simulink library "thc"  (R2021b)
settings: Solver=VariableStepAuto  StartTime=0.0  StopTime=10.0  RelTol=1e-3
undefined symbols (not defined in the file): ATHC_APTCQA_X_C, ATHC_APTCQB_X_C, ATHC_dAy_X_C, ATHC_Qeq_X_kmh, ATHC_VbaseC_X_C, ATHC_VbaseC_Y_W, ATHC_VbaseD_X_C, ATHC_VbaseH_X_C, FALSE, KTHC_ACMaxMinT_sec, KTHC_aDeice_K, KTHC_AGSDefLv_K, KTHC_AGSLv1_K, KTHC_AGSLv2_K, KTHC_AGSLv3_K, KTHC_AGSLv4_K, KTHC_AGSLv5_K, KTHC_AirIntUpdateT_sec, KTHC_APTCOneZoneMax_W, KTHC_APTCPeriod_cnt, KTHC_APTCPWMEN_flg, KTHC_APTCQMaxC_W, KTHC_APTCQminC_W, KTHC_APTCQminD_W, KTHC_APTCQminRe1_W, KTHC_APTCQminRe_W, KTHC_APTCQoffT_cnt, KTHC_APTCQonT_cnt, KTHC_APTCRiLeMaxDff_W, KTHC_APTCRiLeMinDff_W, KTHC_BatCoolT_cnt, KTHC_BatInTempDef_C, KTHC_bDeice_K, KTHC_CompMaxDeice_rpm, KTHC_CompMinDeice_rpm, KTHC_CompSotxvOp_K, KTHC_CompSotxvOpLow_rpm, KTHC_CompSpdmax_rpm, KTHC_CompSpdmaxBC1_rpm, KTHC_CompSpdmaxBC_rpm, KTHC_CompSpdmid1_rpm, KTHC_CompSpdmid2_rpm, KTHC_CompSpdmid3_rpm, KTHC_CompSpdmid_rpm, KTHC_CompSpdmin_rpm, KTHC_DAPTCQ1_W, KTHC_DAPTCQ2_W, KTHC_DAPTCQ3_W, KTHC_DcChSetTemp_C, KTHC_DehumidityEN_flg, KTHC_DeiceCycTime_K, KTHC_DriveLevelWPTCBAH1_W, KTHC_DriveLevelWPTCBAH2_W, KTHC_DriveLevelWPTCBAH3_W, KTHC_DriveLevelWPTCBAH4_W, KTHC_DriverSeatPos_flg, KTHC_DriveT1MinBAH_C, KTHC_DriveT2MaxBAH_C, KTHC_DriveT2MinBAH_C, KTHC_DriveT3MaxBAH_C ... (+379)
libraries: simulink x489
(part 5 of 17)

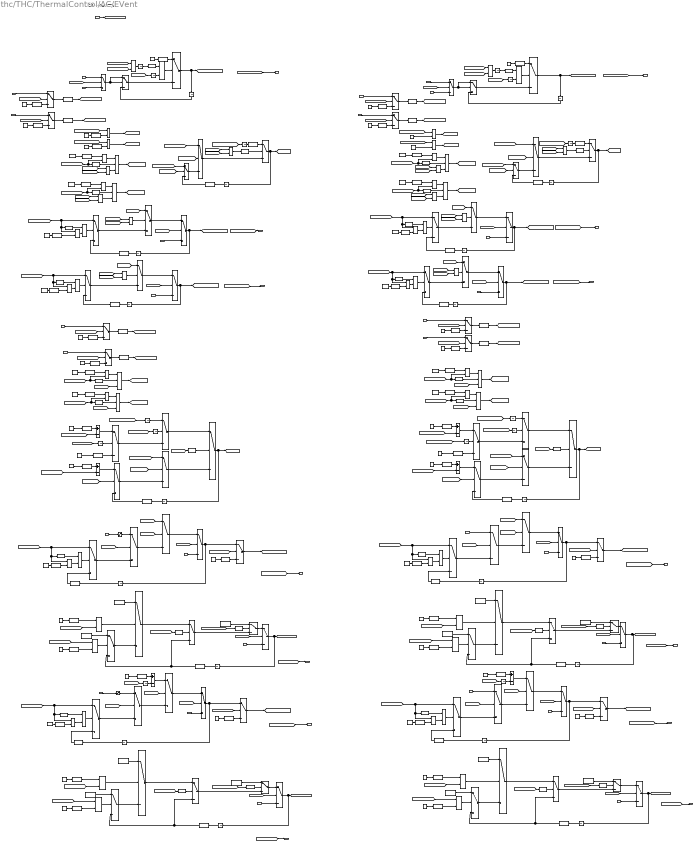
== system thc/THC/ThermalControl/AC/EVent ==
  note: Passenger Side
  note: Driver Side
  fInitial : Inport
  VINP_IVILBlowerModeSta_enum : Inport  Port=2
  VINP_FDCTHCLEventModeStaM_enum : Inport  Port=3
  VINP_IVIRBlowerModeSta_enum : Inport  Port=4
  VINP_FDCTHCREventModeStaM_enum : Inport  Port=5
  VINP_IVILBlowerZSta_enum : Inport  Port=6
  VINP_IVICLBlowerZSta_enum : Inport  Port=7
  VINP_IVIRBlowerZSta_enum : Inport  Port=8
  VINP_IVICRBlowerZSta_enum : Inport  Port=9
  VINP_FDCTHCLEventZStaM_enum : Inport  Port=10
  VINP_FDCTHCCLEVentZStaM_enum : Inport  Port=11
  VINP_FDCTHCREventZStaM_enum : Inport  Port=12
  VINP_FDCTHCCREVentZStaM_enum : Inport  Port=13
  VINP_IVILBlowerYSta_enum : Inport  Port=14
  VINP_IVICLBlowerYSta_enum : Inport  Port=15
  VINP_ZFRTHCLEventActYSta_enum : Inport  Port=16
  VTHC_FDCTHCLVentENM_flg : Inport  Port=17
  VINP_FDCTHCLEventYStaM_enum : Inport  Port=18
  VINP_ZFRTHCCLEVentActYSta_enum : Inport  Port=19
  VTHC_FDCTHCCLVentENM_flg : Inport  Port=20
  VINP_FDCTHCCLEVentYStaM_enum : Inport  Port=21
  VINP_IVIRBlowerYSta_enum : Inport  Port=22
  VINP_IVICRBlowerYSta_enum : Inport  Port=23
  VINP_ZFRTHCREventActYSta_enum : Inport  Port=24
  VTHC_FDCTHCRVentENM_flg : Inport  Port=25
  VINP_FDCTHCREventYStaM_enum : Inport  Port=26
  VINP_ZFRTHCCREVentActYSta_enum : Inport  Port=27
  VTHC_FDCTHCCRVentENM_flg : Inport  Port=28
  VINP_FDCTHCCREVentYStaM_enum : Inport  Port=29
  VINP_CANMsgValidIVI2_flg : Inport  Port=30
  Add{,1..5} (6 alike) : Sum  Inputs=+-
  Constant{,1,4..5,7..8,10,14,18,23,25,28..29,33,38,40..42,45..46,48..51,53..54} (26 alike) : Constant  Value=100
  Constant11 : Constant  Value=3
  Constant12 : Constant  Value=50
  Constant{6,9,13,19,24,34,39,47} (8 alike) : Constant  Value=true
  Constant{15..16,20..21,30..31,35..36} (8 alike) : Constant  Value=126
  Constant{17,22,32,37} (4 alike) : Constant  Value=false
  Constant2 : Constant  Value=2
  Constant26 : Constant  Value=3
  Constant27 : Constant  Value=50
  Constant3 : Constant  Value=2
  Constant43 : Constant
  Constant44 : Constant
  Constant{52,55..61} (8 alike) : Constant  Value=127
  Data Type Conversion{,1..20,22..25,27..35,37..40,42..73} (70 alike) : DataTypeConversion  OutDataTypeStr=uint8
  Data Type Conversion{21,26,36,41} (4 alike) : DataTypeConversion  OutDataTypeStr=boolean
  Detect Change{,1..17,19..20} (20 alike) : simulink/Logic and Bit Operations/Detect Change  vinit=0  OutDataTypeStr=boolean
  Detect Decrease : simulink/Logic and Bit Operations/Detect Decrease  vinit=0.0  OutDataTypeStr=boolean
  Detect Decrease1 : simulink/Logic and Bit Operations/Detect Decrease  vinit=0.0  OutDataTypeStr=boolean
  Detect Increase{,1..7} (8 alike) : simulink/Logic and Bit Operations/Detect Increase  vinit=0.0  OutDataTypeStr=boolean
  Logical Operator{,1..3,5..8} (8 alike) : Logic  Inputs=3  AllPortsSameDT=off  OutDataTypeStr=boolean
  Logical Operator{9..12,22..29} (12 alike) : Logic  AllPortsSameDT=off  OutDataTypeStr=boolean
  Logical Operator{4,13..21} (10 alike) : Logic  Operator=OR  AllPortsSameDT=off  OutDataTypeStr=boolean
  Relational Operator{,1,4..5,7..8,22..23} (8 alike) : RelationalOperator  OutDataTypeStr=boolean  RndMeth=Simplest
  Relational Operator{2,9..10,13,15..16,19,21,24..25,27..28} (12 alike) : RelationalOperator  Operator=<=  OutDataTypeStr=boolean  RndMeth=Simplest
  Relational Operator{3,6,11..12,14,17..18,20} (8 alike) : RelationalOperator  Operator===  OutDataTypeStr=boolean  RndMeth=Simplest
  Saturation : Saturate  UpperLimit=100  LowerLimit=0
  Saturation1 : Saturate  UpperLimit=100  LowerLimit=0
  Switch{,1..81} (82 alike) : Switch  Criteria=u2 > Threshold
  Unit Delay{,1..31} (32 alike) : UnitDelay  SampleTime=-1  HasFrameUpgradeWarning=on
  VTHC_FDCTHCLEventModeSta_enum : Outport
  VTHC_FDCTHCREventModeSta_enum : Outport  Port=2
  VTHC_FDCTHCLEventZSta_enum : Outport  Port=3
  VTHC_FDCTHCCLEVentZSta_enum : Outport  Port=4
  VTHC_FDCTHCREventZSta_enum : Outport  Port=5
  VTHC_FDCTHCCREVentZSta_enum : Outport  Port=6
  VTHC_FDCTHCLEventYSta_enum : Outport  Port=7
  VTHC_FDCTHCLVentEN_flg : Outport  Port=8
  VTHC_FDCTHCCLEVentYSta_enum : Outport  Port=9
  VTHC_FDCTHCCLVentEN_flg : Outport  Port=10
  VTHC_FDCTHCREventYSta_enum : Outport  Port=11
  VTHC_FDCTHCRVentEN_flg : Outport  Port=12
  VTHC_FDCTHCCREVentYSta_enum : Outport  Port=13
  VTHC_FDCTHCCRVentEN_flg : Outport  Port=14
  wires:
  Data Type Conversion73/1 -> Switch81/3
  [VINP_CANMsgValidIVI2_flg] -> Switch81/2
  Switch81/1 -> Data Type Conversion65/1
  VINP_IVICRBlowerYSta_enum/1 -> Switch81/1
  Constant61/1 -> Data Type Conversion73/1
  Constant60/1 -> Data Type Conversion72/1
  VINP_IVIRBlowerYSta_enum/1 -> Switch80/1
  Switch80/1 -> Data Type Conversion64/1
  [VINP_CANMsgValidIVI2_flg] -> Switch80/2
  Data Type Conversion72/1 -> Switch80/3
  VINP_IVICLBlowerYSta_enum/1 -> Switch79/1
  Switch79/1 -> Data Type Conversion63/1
  [VINP_CANMsgValidIVI2_flg] -> Switch79/2
  Constant59/1 -> Data Type Conversion71/1
  Data Type Conversion71/1 -> Switch79/3
  Data Type Conversion70/1 -> Switch78/3
  Constant58/1 -> Data Type Conversion70/1
  [VINP_CANMsgValidIVI2_flg] -> Switch78/2
  Switch78/1 -> Data Type Conversion62/1
  VINP_IVILBlowerYSta_enum/1 -> Switch78/1
  Switch77/1 -> Data Type Conversion61/1
  VINP_IVICRBlowerZSta_enum/1 -> Switch77/1
  [VINP_CANMsgValidIVI2_flg] -> Switch77/2
  Constant57/1 -> Data Type Conversion69/1
  Data Type Conversion69/1 -> Switch77/3
  Data Type Conversion68/1 -> Switch76/3
  Constant56/1 -> Data Type Conversion68/1
  [VINP_CANMsgValidIVI2_flg] -> Switch76/2
  Switch76/1 -> Data Type Conversion60/1
  VINP_IVIRBlowerZSta_enum/1 -> Switch76/1
  VINP_IVICLBlowerZSta_enum/1 -> Switch75/1
  Switch75/1 -> Data Type Conversion59/1
  [VINP_CANMsgValidIVI2_flg] -> Switch75/2
  Constant55/1 -> Data Type Conversion67/1
  Data Type Conversion67/1 -> Switch75/3
  Data Type Conversion66/1 -> Switch74/3
  Constant52/1 -> Data Type Conversion66/1
  [VINP_CANMsgValidIVI2_flg] -> Switch74/2
  Switch74/1 -> Data Type Conversion56/1
  VINP_CANMsgValidIVI2_flg/1 -> [VINP_CANMsgValidIVI2_flg]
  Logical Operator29/1 -> Switch15/2
  [VINP_IVILBlowerZSta_enum] -> Switch12/1, Detect Change13/1, Relational Operator9/1
  Relational Operator9/1 -> Logical Operator28/2
  Detect Change13/1 -> Logical Operator28/1
  Logical Operator28/1 -> Switch12/2
  Logical Operator27/1 -> Switch21/2
  Relational Operator10/1 -> Logical Operator26/2
  [VTHC_FDCTHCCLEVentYSta_enum] -> Add/2
  Constant14/1 -> Data Type Conversion19/1
  Data Type Conversion19/1 -> Add1/1
  [VINP_IVILBlowerYSta_enum] -> Relational Operator13/1
  [fInitial] -> Switch44/2
  VINP_FDCTHCREventYStaM_enum/1 -> Switch58/3
  Constant39/1 -> Switch66/1
  VINP_FDCTHCCREVentYStaM_enum/1 -> Switch67/3
  [VINP_IVICRBlowerYSta_enum] -> Relational Operator23/2, Detect Change9/1
  Relational Operator23/1 -> Logical Operator8/1
  [VTHC_FDCTHCRVentEN_flg] -> Unit Delay26/1
  Data Type Conversion45/1 -> Relational Operator22/1
  Relational Operator7/1 -> Logical Operator5/1
  Detect Change5/1 -> Logical Operator6/2
  Logical Operator6/1 -> [CLYupdate]
  Data Type Conversion21/1 -> Switch32/3, Switch34/3
  VINP_FDCTHCCLEVentYStaM_enum/1 -> Switch44/3
  Switch35/1 -> Switch30/1, Unit Delay11/1
  Switch33/1 -> Switch32/1
  [fInitial] -> Switch35/2
  [VTHC_FDCTHCLVentEN_flg] -> VTHC_FDCTHCLVentEN_flg/1
  Relational Operator14/1 -> Switch42/2
  Switch43/1 -> Switch42/3
  Constant23/1 -> Data Type Conversion29/1
  Logical Operator15/1 -> Switch10/2
  [VTHC_FDCTHCLEventYSta_enum] -> VTHC_FDCTHCLEventYSta_enum/1
  Data Type Conversion23/1 -> Relational Operator12/1
  [fInitial] -> Switch63/2
  Constant26/1 -> Relational Operator17/2
  [VTHC_FDCTHCREventModeSta_enum] -> Relational Operator17/1
  Constant8/1 -> Data Type Conversion7/1
  Data Type Conversion41/1 -> Switch66/3, Switch64/3
  VTHC_FDCTHCCRVentENM_flg/1 -> Switch63/3
  [VTHC_FDCTHCLVentEN_flg] -> Switch30/2
  [LBalanceZ] -> Switch13/1
  [LBalanceMode] -> Detect Increase2/1
  Switch12/1 -> Switch10/3
  Constant19/1 -> Switch34/1
  Logical Operator16/1 -> Switch13/2
  VINP_FDCTHCCLEVentZStaM_enum/1 -> Switch14/3
  Switch15/1 -> Switch13/3
  Switch13/1 -> Switch14/1
  Switch10/1 -> Switch11/1
  Relational Operator18/1 -> Switch56/2
  Relational Operator4/1 -> Logical Operator2/1
  Data Type Conversion62/1 -> [VINP_IVILBlowerYSta_enum]
  Constant5/1 -> Data Type Conversion3/1
  Data Type Conversion3/1 -> Relational Operator5/1
  Constant4/1 -> Data Type Conversion2/1
  Switch28/1 -> Switch27/3
  Detect Change3/1 -> Logical Operator3/2
  Logical Operator3/1 -> [CRZupdate]
  Switch8/1 -> Switch9/3
  Logical Operator2/1 -> [RZupdate]
  [CRZupdate] -> Switch7/2
  Detect Increase1/1 -> Switch9/2
  Switch9/1 -> Unit Delay3/1, [RBalanceZ]
  Unit Delay3/1 -> Data Type Conversion5/1
  Data Type Conversion61/1 -> [VINP_IVICRBlowerZSta_enum]
  [VINP_IVIRBlowerZSta_enum] -> Detect Change2/1, Relational Operator4/2
  Constant7/1 -> Data Type Conversion6/1
  Data Type Conversion11/1 -> Switch15/3
  [LSweepMode] -> Switch28/2
  Switch24/1 -> Switch23/3
  Data Type Conversion9/1 -> Switch9/1
  Unit Delay12/1 -> Data Type Conversion21/1
  Logical Operator5/1 -> [LYupdate]
  Switch48/1 -> Switch47/3
  Switch36/1 -> Switch44/1
  Switch22/1 -> Switch23/1
  Logical Operator13/1 -> Logical Operator1/3
  [VTHC_FDCTHCCREVentZSta_enum] -> VTHC_FDCTHCCREVentZSta_enum/1
  Switch40/1 -> Unit Delay14/1, [VTHC_FDCTHCCLVentEN_flg]
  VTHC_FDCTHCCLVentENM_flg/1 -> Switch40/3
  [LBalanceY] -> Switch27/1
  Data Type Conversion5/1 -> Switch7/3
  [LBalanceMode] -> Switch36/2
  [LSweepMode] -> Switch37/2
  Switch38/1 -> Switch37/3
  Switch37/1 -> Switch36/3
  Switch44/1 -> Unit Delay13/1, Switch39/1
  Data Type Conversion25/1 -> Switch38/3
  Switch39/1 -> [VTHC_FDCTHCCLEVentYSta_enum]
  Switch63/1 -> Unit Delay18/1, [VTHC_FDCTHCCRVentEN_flg]
  Unit Delay13/1 -> Data Type Conversion25/1
  Data Type Conversion4/1 -> Switch4/3
  Switch6/1 -> [LBalanceZ], Unit Delay2/1
  [CRYupdate] -> Switch48/2
  Constant27/1 -> Data Type Conversion32/1
  Data Type Conversion32/1 -> Switch49/3
  Constant32/1 -> Switch56/1
  Unit Delay27/1 -> Switch49/2
  Unit Delay17/1 -> Data Type Conversion40/1
  Switch52/1 -> Switch51/3
  Switch67/1 -> Unit Delay17/1, Switch62/1
  Constant31/1 -> Data Type Conversion37/1
  Data Type Conversion30/1 -> Switch48/3
  Unit Delay15/1 -> Data Type Conversion35/1
  Switch57/1 -> Switch56/3
  [VTHC_FDCTHCCREVentYSta_enum] -> VTHC_FDCTHCCREVentYSta_enum/1
  Data Type Conversion37/1 -> Switch53/3
  Relational Operator21/1 -> Switch66/2
  [VTHC_FDCTHCCRVentEN_flg] -> Switch62/2
  [VINP_IVIRBlowerYSta_enum] -> Relational Operator18/2
  Constant30/1 -> Data Type Conversion38/1
  Constant36/1 -> Data Type Conversion42/1
  [RBalanceY] -> Switch50/1
  Data Type Conversion13/1 -> Switch21/3
  Detect Change10/1 -> Switch55/2
  [RBalanceMode] -> Switch59/2
  Switch54/1 -> Unit Delay16/1, [VTHC_FDCTHCRVentEN_flg]
  Constant33/1 -> Data Type Conversion39/1
  Data Type Conversion33/1 -> Add2/1
  Data Type Conversion6/1 -> Relational Operator7/1
  [RSweepMode] -> Switch60/2
  Switch60/1 -> Switch59/3
  Data Type Conversion40/1 -> Switch61/3
  VINP_ZFRTHCREventActYSta_enum/1 -> Switch51/1
  VTHC_FDCTHCRVentENM_flg/1 -> Switch54/3
  Unit Delay1/1 -> Switch2/3
  VINP_FDCTHCREventModeStaM_enum/1 -> Switch3/3
  fInitial/1 -> [fInitial]
  Detect Change2/1 -> Logical Operator2/2
  [VINP_IVICLBlowerZSta_enum] -> Detect Change1/1, Relational Operator1/2
  [VINP_IVICLBlowerYSta_enum] -> Relational Operator8/2, Detect Change5/1
  Data Type Conversion1/1 -> Relational Operator1/1
  Constant1/1 -> Data Type Conversion1/1
  VINP_ZFRTHCCLEVentActYSta_enum/1 -> Saturation/1
  Constant34/1 -> Switch57/1
  [VINP_IVILBlowerZSta_enum] -> Switch5/1
  [VINP_IVILBlowerYSta_enum] -> Detect Change6/1
  Switch5/1 -> Switch6/3
  Constant/1 -> Data Type Conversion/1
  Detect Change/1 -> Logical Operator/2
  Data Type Conversion26/1 -> Switch43/3, Switch41/3
  [CLZupdate] -> Switch4/2
  Unit Delay18/1 -> Data Type Conversion41/1
  Switch14/1 -> [VTHC_FDCTHCCLEVentZSta_enum], Unit Delay5/1
  Relational Operator17/1 -> [RBalanceMode]
  Unit Delay6/1 -> Data Type Conversion12/1
  [VINP_IVICRBlowerYSta_enum] -> Add3/2
  Unit Delay7/1 -> Data Type Conversion13/1
  Switch18/1 -> Switch16/3
  [VINP_IVICLBlowerYSta_enum] -> Detect Change7/1
  VINP_FDCTHCCREVentZStaM_enum/1 -> Switch20/3
  [fInitial] -> Switch20/2
  [RBalanceMode] -> Logical Operator8/3
  Switch19/1 -> Switch20/1
  Logical Operator20/1 -> Switch19/2
  Switch21/1 -> Switch19/3
  [fInitial] -> Switch11/2
  VINP_ZFRTHCLEventActYSta_enum/1 -> Saturation1/1
  Relational Operator6/1 -> [LSweepMode]
  VINP_FDCTHCLEventModeStaM_enum/1 -> Switch1/3
  Constant20/1 -> Data Type Conversion28/1
  Unit Delay4/1 -> Data Type Conversion10/1
  Switch29/1 -> Switch28/3
  Constant18/1 -> Data Type Conversion24/1
  Logical Operator/1 -> [LZupdate]
  Data Type Conversion60/1 -> [VINP_IVIRBlowerZSta_enum]
  Switch4/1 -> Switch5/3
  Data Type Conversion18/1 -> Add/1
  Switch26/1 -> Switch22/3
  [VTHC_FDCTHCREventZSta_enum] -> Unit Delay9/1
  Relational Operator/1 -> Logical Operator/1
  [VTHC_FDCTHCLEventZSta_enum] -> VTHC_FDCTHCLEventZSta_enum/1
  [CLYupdate] -> Switch25/2
  Unit Delay5/1 -> Data Type Conversion11/1
  Data Type Conversion16/1 -> Switch26/3
  Constant17/1 -> Switch33/1
  Detect Increase3/1 -> Switch46/2
  Unit Delay9/1 -> Data Type Conversion9/1
  [VTHC_FDCTHCCLVentEN_flg] -> Unit Delay24/1
  Data Type Conversion34/1 -> Add3/1
  Detect Change9/1 -> Logical Operator8/2
  Switch62/1 -> [VTHC_FDCTHCCREVentYSta_enum]
  Switch46/1 -> [RBalanceY], Unit Delay19/1
  [VINP_IVIRBlowerYSta_enum] -> Switch47/1
  [VTHC_FDCTHCCRVentEN_flg] -> VTHC_FDCTHCCRVentEN_flg/1
  Add3/1 -> Switch48/1
  [RBalanceMode] -> Logical Operator7/3
  Detect Change6/1 -> Switch32/2
  [VTHC_FDCTHCCREVentYSta_enum] -> Add2/2
  Data Type Conversion28/1 -> Relational Operator14/1
  [fInitial] -> Switch54/2
  Switch50/1 -> Switch58/1
  [RYupdate] -> Switch47/2
  Constant25/1 -> Data Type Conversion33/1
  [VINP_IVICRBlowerZSta_enum] -> Relational Operator5/2, Detect Change3/1
  Switch32/1 -> Switch70/3
  [VINP_IVILBlowerZSta_enum] -> Relational Operator/2, Detect Change/1
  Logical Operator1/1 -> [CLZupdate]
  Data Type Conversion17/1 -> Switch6/1
  [VTHC_FDCTHCLEventZSta_enum] -> Unit Delay10/1
  Data Type Conversion42/1 -> Switch62/3
  [LBalanceZ] -> Switch10/1
  Unit Delay14/1 -> Data Type Conversion26/1
  VINP_IVIRBlowerModeSta_enum/1 -> Switch3/1
  Logical Operator8/1 -> [CRYupdate]
  [VTHC_FDCTHCREventModeSta_enum] -> VTHC_FDCTHCREventModeSta_enum/1
  Constant11/1 -> Data Type Conversion50/1
  Relational Operator13/1 -> Switch34/2
  VINP_IVILBlowerModeSta_enum/1 -> Switch1/1
  Switch1/1 -> Switch/1, Switch/2
  [fInitial] -> Switch3/2
  VTHC_FDCTHCLVentENM_flg/1 -> Switch31/3
  [VTHC_FDCTHCCLEVentZSta_enum] -> VTHC_FDCTHCCLEVentZSta_enum/1
  Switch27/1 -> Switch35/1
  [VTHC_FDCTHCLEventModeSta_enum] -> Relational Operator11/1
  Data Type Conversion24/1 -> Relational Operator13/2
  [VINP_IVICLBlowerYSta_enum] -> Relational Operator15/1
  [fInitial] -> Switch14/2
  Switch25/1 -> Switch24/3
  Unit Delay2/1 -> Data Type Conversion4/1
  Relational Operator1/1 -> Logical Operator1/1
  [VINP_IVILBlowerYSta_enum] -> Switch24/1
  [VINP_IVICRBlowerYSta_enum] -> Relational Operator21/1
  Logical Operator19/1 -> Switch16/2
  VINP_FDCTHCREventZStaM_enum/1 -> Switch17/3
  Detect Change4/1 -> Logical Operator5/2
  [fInitial] -> Switch17/2
  Switch17/1 -> [VTHC_FDCTHCREventZSta_enum], Unit Delay6/1
  [VINP_IVILBlowerYSta_enum] -> Detect Change4/1, Relational Operator7/2
  Switch16/1 -> Switch17/1
  Data Type Conversion20/1 -> Switch29/3
  Data Type Conversion27/1 -> Switch39/3
  [VTHC_FDCTHCREventModeSta_enum] -> Relational Operator3/1
  Constant3/1 -> Relational Operator3/2
  Relational Operator3/1 -> [RSweepMode]
  [VTHC_FDCTHCCLVentEN_flg] -> Switch39/2
  [VTHC_FDCTHCCLEVentYSta_enum] -> VTHC_FDCTHCCLEVentYSta_enum/1
  Constant2/1 -> Data Type Conversion49/1
  [VTHC_FDCTHCLEventModeSta_enum] -> Relational Operator6/1
  [VTHC_FDCTHCRVentEN_flg] -> Switch53/2
  [RBalanceMode] -> Detect Increase3/1
  Switch41/1 -> Switch71/3
  [RSweepMode] -> Switch51/2
  Switch45/1 -> Switch46/1
  Logical Operator7/1 -> [RYupdate]
  Constant12/1 -> Data Type Conversion16/1
  Switch3/1 -> Switch2/2, Switch2/1
  Switch47/1 -> Switch46/3
  Switch11/1 -> Unit Delay4/1, [VTHC_FDCTHCLEventZSta_enum]
  Data Type Conversion35/1 -> Switch52/3
  Switch59/1 -> Switch67/1
  Data Type Conversion7/1 -> Relational Operator8/1
  Detect Change11/1 -> Switch64/2
  Add2/1 -> Switch49/1
  Relational Operator19/1 -> Switch57/2
  [VINP_IVIRBlowerYSta_enum] -> Detect Change8/1, Relational Operator22/2
  [VINP_IVIRBlowerZSta_enum] -> Switch8/1
  Switch53/1 -> [VTHC_FDCTHCREventYSta_enum]
  [VINP_IVIRBlowerYSta_enum] -> Relational Operator19/1
  [fInitial] -> Switch67/2
  Relational Operator22/1 -> Logical Operator7/1
  Switch20/1 -> Unit Delay7/1, [VTHC_FDCTHCCREVentZSta_enum]
  Constant41/1 -> Data Type Conversion46/1
  Constant40/1 -> Data Type Conversion45/1
  [VTHC_FDCTHCLEventModeSta_enum] -> VTHC_FDCTHCLEventModeSta_enum/1
  [VINP_IVICRBlowerZSta_enum] -> Switch7/1
  Unit Delay10/1 -> Data Type Conversion17/1
  Detect Increase/1 -> Switch6/2
  [LZupdate] -> Switch5/2
  Detect Change8/1 -> Logical Operator7/2
  Switch58/1 -> Switch53/1, Unit Delay15/1
  Switch30/1 -> [VTHC_FDCTHCLEventYSta_enum]
  [VTHC_FDCTHCREventYSta_enum] -> Unit Delay31/1
  Add/1 -> Switch26/1
  Detect Change7/1 -> Switch41/2
  [RZupdate] -> Switch8/2
  [fInitial] -> Switch58/2
  Data Type Conversion43/1 -> Relational Operator20/1
  Constant35/1 -> Data Type Conversion43/1
  Relational Operator20/1 -> Switch65/2
  Switch65/1 -> Switch64/1
  Constant38/1 -> Data Type Conversion44/1
  Data Type Conversion46/1 -> Relational Operator23/1
  Data Type Conversion38/1 -> Relational Operator18/1
  [VINP_IVICRBlowerYSta_enum] -> Relational Operator20/2
  [RBalanceMode] -> Switch50/2
  [VTHC_FDCTHCCLVentEN_flg] -> VTHC_FDCTHCCLVentEN_flg/1
  Add1/1 -> Switch25/1
  Unit Delay19/1 -> Data Type Conversion30/1
  Relational Operator15/1 -> Switch43/2
  Switch51/1 -> Switch50/3
  Switch42/1 -> Switch41/1
  Constant24/1 -> Switch43/1
  Data Type Conversion59/1 -> [VINP_IVICLBlowerZSta_enum]
  Unit Delay11/1 -> Data Type Conversion20/1
  Constant15/1 -> Data Type Conversion23/1
  Switch61/1 -> Switch60/3
  [VTHC_FDCTHCREventYSta_enum] -> VTHC_FDCTHCREventYSta_enum/1
  Constant21/1 -> Data Type Conversion27/1
  VINP_FDCTHCLEventZStaM_enum/1 -> Switch11/3
  [RBalanceZ] -> Switch16/1
  Unit Delay16/1 -> Data Type Conversion36/1
  Data Type Conversion14/1 -> Switch25/3
  [VINP_IVILBlowerYSta_enum] -> Relational Operator12/2
  Switch66/1 -> Switch65/3
  Switch56/1 -> Switch55/1
  Unit Delay/1 -> Switch/3
  Constant10/1 -> Data Type Conversion18/1
  Switch49/1 -> Switch45/3
  Switch34/1 -> Switch33/3
  [fInitial] -> Switch31/2
  [RBalanceZ] -> Switch19/1
  [LYupdate] -> Switch24/2
  [VINP_IVICRBlowerYSta_enum] -> Detect Change11/1
  [LBalanceMode] -> Switch27/2
  Relational Operator12/1 -> Switch33/2
  [VINP_IVICLBlowerZSta_enum] -> Switch4/1
  [VINP_IVIRBlowerYSta_enum] -> Detect Change10/1
  Data Type Conversion29/1 -> Relational Operator15/2
  [LBalanceMode] -> Logical Operator5/3
  Detect Change1/1 -> Logical Operator1/2
  [VTHC_FDCTHCRVentEN_flg] -> VTHC_FDCTHCRVentEN_flg/1
  Constant16/1 -> Data Type Conversion22/1
  Data Type Conversion22/1 -> Switch30/3
  Switch7/1 -> Switch8/3
  Data Type Conversion36/1 -> Switch55/3, Switch57/3
  [VINP_IVICLBlowerYSta_enum] -> Relational Operator14/2
  Data Type Conversion12/1 -> Switch18/3
  VINP_IVILBlowerZSta_enum/1 -> Switch74/1
  [fInitial] -> Switch40/2
  Data Type Conversion/1 -> Relational Operator/1
  Data Type Conversion63/1 -> [VINP_IVICLBlowerYSta_enum]
  Switch23/1 -> [LBalanceY], Unit Delay8/1
  Data Type Conversion64/1 -> [VINP_IVIRBlowerYSta_enum]
  Relational Operator8/1 -> Logical Operator6/1
  [VINP_IVICLBlowerYSta_enum] -> Add1/2
  Relational Operator5/1 -> Logical Operator3/1
  Data Type Conversion39/1 -> Relational Operator19/2
  Data Type Conversion44/1 -> Relational Operator21/2
  Switch68/1 -> Unit Delay/1, [VTHC_FDCTHCLEventModeSta_enum]
  VINP_ZFRTHCCREVentActYSta_enum/1 -> Switch60/1
  [VTHC_FDCTHCREventZSta_enum] -> VTHC_FDCTHCREventZSta_enum/1
  Data Type Conversion2/1 -> Relational Operator4/1
  Constant22/1 -> Switch42/1
  [fInitial] -> Switch1/2
  Constant37/1 -> Switch65/1
  Switch31/1 -> [VTHC_FDCTHCLVentEN_flg], Unit Delay12/1
  Data Type Conversion10/1 -> Switch12/3
  Unit Delay8/1 -> Data Type Conversion14/1
  VINP_FDCTHCLEventYStaM_enum/1 -> Switch35/3
  Constant29/1 -> Data Type Conversion34/1
  [LBalanceMode] -> Logical Operator6/3
  [VTHC_FDCTHCCLVentEN_flg] -> Logical Operator9/2
  [VTHC_FDCTHCLVentEN_flg] -> Logical Operator9/1
  Logical Operator9/1 -> Unit Delay20/1
  Unit Delay20/1 -> Detect Decrease/1
  Detect Decrease/1 -> Logical Operator10/1
  Data Type Conversion49/1 -> Relational Operator6/2
  Data Type Conversion50/1 -> Relational Operator11/2
  [LBalanceMode] -> Unit Delay21/1
  Unit Delay21/1 -> Logical Operator10/2
  Logical Operator10/1 -> Switch68/2
  Data Type Conversion51/1 -> Switch68/1
  Constant43/1 -> Data Type Conversion51/1
  Switch/1 -> Switch68/3
  Constant44/1 -> Data Type Conversion52/1
  Data Type Conversion52/1 -> Switch69/1
  Logical Operator11/1 -> Switch69/2
  Detect Decrease1/1 -> Logical Operator11/1
  Unit Delay22/1 -> Detect Decrease1/1
  Logical Operator12/1 -> Unit Delay22/1
  [VTHC_FDCTHCRVentEN_flg] -> Logical Operator12/1
  [VTHC_FDCTHCCRVentEN_flg] -> Logical Operator12/2
  Switch69/1 -> Unit Delay1/1, [VTHC_FDCTHCREventModeSta_enum]
  Switch2/1 -> Switch69/3
  [RBalanceMode] -> Unit Delay23/1
  Unit Delay23/1 -> Logical Operator11/2
  Constant45/1 -> Data Type Conversion53/1
  Data Type Conversion53/1 -> Add4/1
  [LBalanceY] -> Unit Delay28/1
  Add4/1 -> Switch36/1
  Add5/1 -> Switch59/1
  Constant46/1 -> Data Type Conversion54/1
  Data Type Conversion54/1 -> Add5/1
  [RBalanceY] -> Unit Delay30/1
  Logical Operator4/1 -> Logical Operator/3
  [LBalanceMode] -> Logical Operator4/1
  [LSweepMode] -> Logical Operator4/2
  [LSweepMode] -> Logical Operator13/2
  [LBalanceMode] -> Logical Operator13/1
  [LBalanceMode] -> Logical Operator14/1
  [LSweepMode] -> Logical Operator14/2
  Logical Operator14/1 -> Detect Increase/1
  [LBalanceMode] -> Logical Operator15/1
  [LSweepMode] -> Logical Operator15/2
  [LSweepMode] -> Logical Operator16/2
  [LBalanceMode] -> Logical Operator16/1
  Logical Operator17/1 -> Logical Operator2/3
  [RSweepMode] -> Logical Operator17/1
  [RBalanceMode] -> Logical Operator17/2
  [RBalanceMode] -> Logical Operator18/2
  [RSweepMode] -> Logical Operator18/1
  Logical Operator18/1 -> Logical Operator3/3
  [RSweepMode] -> Logical Operator19/1
  [RBalanceMode] -> Logical Operator19/2
  [RBalanceMode] -> Logical Operator20/2
  [RSweepMode] -> Logical Operator20/1
  [RBalanceMode] -> Logical Operator21/2
  [RSweepMode] -> Logical Operator21/1
  Logical Operator21/1 -> Detect Increase1/1
  Switch70/1 -> Switch31/1
  Constant6/1 -> Switch70/1
  Detect Increase5/1 -> Switch70/2
  [LBalanceMode] -> Detect Increase5/1
  [LBalanceMode] -> Detect Increase4/1
  Detect Increase4/1 -> Switch71/2
  Constant47/1 -> Switch71/1
  Switch71/1 -> Switch40/1
  [VTHC_FDCTHCLEventYSta_enum] -> Unit Delay29/1
  Detect Increase2/1 -> Switch23/2
  Saturation/1 -> Switch37/1
  Saturation1/1 -> Switch28/1
  Unit Delay24/1 -> Switch26/2
  [VTHC_FDCTHCLVentEN_flg] -> Unit Delay25/1
  Unit Delay25/1 -> Switch22/2
  Unit Delay26/1 -> Switch45/2
  [VTHC_FDCTHCCRVentEN_flg] -> Unit Delay27/1
  [RBalanceMode] -> Detect Increase7/1
  Detect Increase7/1 -> Switch72/2
  Constant9/1 -> Switch72/1
  Switch55/1 -> Switch72/3
  Switch72/1 -> Switch54/1
  Switch64/1 -> Switch73/3
  Constant13/1 -> Switch73/1
  Detect Increase6/1 -> Switch73/2
  [RBalanceMode] -> Detect Increase6/1
  Switch73/1 -> Switch63/1
  [VINP_IVICLBlowerZSta_enum] -> Switch15/1, Detect Change12/1, Relational Operator2/1
  Detect Change12/1 -> Logical Operator29/1
  Data Type Conversion8/1 -> Relational Operator2/2
  Constant28/1 -> Data Type Conversion8/1
  Relational Operator2/1 -> Logical Operator29/2
  Constant42/1 -> Data Type Conversion15/1
  Data Type Conversion15/1 -> Relational Operator9/2
  [VINP_IVIRBlowerZSta_enum] -> Switch18/1, Relational Operator10/1, Detect Change14/1
  Detect Change14/1 -> Logical Operator26/1
  Data Type Conversion31/1 -> Relational Operator10/2
  Constant48/1 -> Data Type Conversion31/1
  Logical Operator26/1 -> Switch18/2
  Relational Operator16/1 -> Logical Operator27/2
  Constant49/1 -> Data Type Conversion47/1
  Data Type Conversion47/1 -> Relational Operator16/2
  Detect Change15/1 -> Logical Operator27/1
  [VINP_IVICRBlowerZSta_enum] -> Relational Operator16/1, Detect Change15/1, Switch21/1
  Constant51/1 -> Data Type Conversion55/1
  Data Type Conversion55/1 -> Relational Operator25/2
  Detect Change17/1 -> Logical Operator22/1
  [VINP_IVICRBlowerYSta_enum] -> Switch61/1, Relational Operator25/1, Detect Change17/1
  Relational Operator25/1 -> Logical Operator22/2
  Logical Operator24/1 -> Switch29/2
  Logical Operator22/1 -> Switch61/2
  Logical Operator23/1 -> Switch52/2
  Relational Operator28/1 -> Logical Operator23/2
  [VINP_IVIRBlowerYSta_enum] -> Switch52/1, Detect Change20/1, Relational Operator28/1
  Detect Change20/1 -> Logical Operator23/1
  Data Type Conversion58/1 -> Relational Operator28/2
  Constant54/1 -> Data Type Conversion58/1
  Constant50/1 -> Data Type Conversion48/1
  Data Type Conversion48/1 -> Relational Operator24/2
  Detect Change16/1 -> Logical Operator24/1
  [VINP_IVILBlowerYSta_enum] -> Switch29/1, Relational Operator24/1, Detect Change16/1
  Relational Operator24/1 -> Logical Operator24/2
  Relational Operator27/1 -> Logical Operator25/2
  [VINP_IVICLBlowerYSta_enum] -> Detect Change19/1, Relational Operator27/1, Switch38/1
  Detect Change19/1 -> Logical Operator25/1
  Data Type Conversion57/1 -> Relational Operator27/2
  Constant53/1 -> Data Type Conversion57/1
  Logical Operator25/1 -> Switch38/2
  Relational Operator11/1 -> [LBalanceMode]
  Unit Delay28/1 -> Add4/2
  Unit Delay29/1 -> Switch22/1
  Unit Delay30/1 -> Add5/2
  Unit Delay31/1 -> Switch45/1
  Data Type Conversion56/1 -> [VINP_IVILBlowerZSta_enum]
  Data Type Conversion65/1 -> [VINP_IVICRBlowerYSta_enum]

== system thc/THC/ThermalControl/AC/HMISwitchReceive ==
  VINP_HMIZLSetTPCmd_flg : Inport
  Add : Sum
  Bitwise AND : simulink/Logic and Bit Operations/Bitwise Operator  logicop=AND  UseBitMask=on  BitMask=bin2dec('1')  BitMaskRealWorld=Stored Integer
  Compare To Constant : simulink/Logic and Bit Operations/Compare To Constant  relop=>  const=11  OutDataTypeStr=boolean
  Constant : Constant  Value=0
  Constant1 : Constant
  Data Type Conversion : DataTypeConversion  OutDataTypeStr=uint8
  Data Type Conversion1 : DataTypeConversion  OutDataTypeStr=uint8
  Data Type Conversion2 : DataTypeConversion  OutDataTypeStr=boolean
  Detect Increase : simulink/Logic and Bit Operations/Detect Increase  vinit=0.0  OutDataTypeStr=boolean
  Logical Operator : Logic  Operator=OR  AllPortsSameDT=off  OutDataTypeStr=boolean
  Logical Operator1 : Logic  AllPortsSameDT=off  OutDataTypeStr=boolean
  Switch : Switch  Criteria=u2 > Threshold
  Unit Delay : UnitDelay  SampleTime=-1  HasFrameUpgradeWarning=on
  Out1 : Outport
  wires:
  Constant/1 -> Data Type Conversion/1
  Data Type Conversion/1 -> Switch/3
  Add/1 -> Switch/1
  Switch/1 -> Unit Delay/1, Bitwise AND/1, Compare To Constant/1
  Bitwise AND/1 -> Data Type Conversion2/1
  Data Type Conversion1/1 -> Add/2
  VINP_HMIZLSetTPCmd_flg/1 -> Switch/2, Detect Increase/1
  Logical Operator1/1 -> Logical Operator/1
  Detect Increase/1 -> Logical Operator/2
  Unit Delay/1 -> Add/1
  Constant1/1 -> Data Type Conversion1/1
  Logical Operator/1 -> Out1/1
  Compare To Constant/1 -> Logical Operator1/1
  Data Type Conversion2/1 -> Logical Operator1/2

== system thc/THC/ThermalControl/AC/HMISwitchReceive1 ==
  VINP_HMIZLSetTMCmd_flg : Inport
  Add : Sum
  Bitwise AND : simulink/Logic and Bit Operations/Bitwise Operator  logicop=AND  UseBitMask=on  BitMask=bin2dec('1')  BitMaskRealWorld=Stored Integer
  Compare To Constant : simulink/Logic and Bit Operations/Compare To Constant  relop=>  const=11  OutDataTypeStr=boolean
  Constant : Constant  Value=0
  Constant1 : Constant
  Data Type Conversion : DataTypeConversion  OutDataTypeStr=uint8
  Data Type Conversion1 : DataTypeConversion  OutDataTypeStr=uint8
  Data Type Conversion2 : DataTypeConversion  OutDataTypeStr=boolean
  Detect Increase : simulink/Logic and Bit Operations/Detect Increase  vinit=0.0  OutDataTypeStr=boolean
  Logical Operator : Logic  Operator=OR  AllPortsSameDT=off  OutDataTypeStr=boolean
  Logical Operator1 : Logic  AllPortsSameDT=off  OutDataTypeStr=boolean
  Switch : Switch  Criteria=u2 > Threshold
  Unit Delay : UnitDelay  SampleTime=-1  HasFrameUpgradeWarning=on
  Out1 : Outport
  wires:
  Data Type Conversion2/1 -> Logical Operator1/2
  Compare To Constant/1 -> Logical Operator1/1
  Logical Operator/1 -> Out1/1
  Constant1/1 -> Data Type Conversion1/1
  Unit Delay/1 -> Add/1
  Detect Increase/1 -> Logical Operator/2
  Logical Operator1/1 -> Logical Operator/1
  VINP_HMIZLSetTMCmd_flg/1 -> Detect Increase/1, Switch/2
  Data Type Conversion1/1 -> Add/2
  Bitwise AND/1 -> Data Type Conversion2/1
  Switch/1 -> Compare To Constant/1, Bitwise AND/1, Unit Delay/1
  Add/1 -> Switch/1
  Data Type Conversion/1 -> Switch/3
  Constant/1 -> Data Type Conversion/1

== system thc/THC/ThermalControl/AC/HMISwitchReceive2 ==
  VINP_HMIZRSetTPCmd_flg : Inport
  Add : Sum
  Bitwise AND : simulink/Logic and Bit Operations/Bitwise Operator  logicop=AND  UseBitMask=on  BitMask=bin2dec('1')  BitMaskRealWorld=Stored Integer
  Compare To Constant : simulink/Logic and Bit Operations/Compare To Constant  relop=>  const=11  OutDataTypeStr=boolean
  Constant : Constant  Value=0
  Constant1 : Constant
  Data Type Conversion : DataTypeConversion  OutDataTypeStr=uint8
  Data Type Conversion1 : DataTypeConversion  OutDataTypeStr=uint8
  Data Type Conversion2 : DataTypeConversion  OutDataTypeStr=boolean
  Detect Increase : simulink/Logic and Bit Operations/Detect Increase  vinit=0.0  OutDataTypeStr=boolean
  Logical Operator : Logic  Operator=OR  AllPortsSameDT=off  OutDataTypeStr=boolean
  Logical Operator1 : Logic  AllPortsSameDT=off  OutDataTypeStr=boolean
  Switch : Switch  Criteria=u2 > Threshold
  Unit Delay : UnitDelay  SampleTime=-1  HasFrameUpgradeWarning=on
  Out1 : Outport
  wires:
  Constant/1 -> Data Type Conversion/1
  Data Type Conversion/1 -> Switch/3
  Add/1 -> Switch/1
  Switch/1 -> Unit Delay/1, Bitwise AND/1, Compare To Constant/1
  Bitwise AND/1 -> Data Type Conversion2/1
  Data Type Conversion1/1 -> Add/2
  VINP_HMIZRSetTPCmd_flg/1 -> Switch/2, Detect Increase/1
  Logical Operator1/1 -> Logical Operator/1
  Detect Increase/1 -> Logical Operator/2
  Unit Delay/1 -> Add/1
  Constant1/1 -> Data Type Conversion1/1
  Logical Operator/1 -> Out1/1
  Compare To Constant/1 -> Logical Operator1/1
  Data Type Conversion2/1 -> Logical Operator1/2

== system thc/THC/ThermalControl/AC/HMISwitchReceive3 ==
  VINP_HMIZRSetTMCmd_flg : Inport
  Add : Sum
  Bitwise AND : simulink/Logic and Bit Operations/Bitwise Operator  logicop=AND  UseBitMask=on  BitMask=bin2dec('1')  BitMaskRealWorld=Stored Integer
  Compare To Constant : simulink/Logic and Bit Operations/Compare To Constant  relop=>  const=11  OutDataTypeStr=boolean
  Constant : Constant  Value=0
  Constant1 : Constant
  Data Type Conversion : DataTypeConversion  OutDataTypeStr=uint8
  Data Type Conversion1 : DataTypeConversion  OutDataTypeStr=uint8
  Data Type Conversion2 : DataTypeConversion  OutDataTypeStr=boolean
  Detect Increase : simulink/Logic and Bit Operations/Detect Increase  vinit=0.0  OutDataTypeStr=boolean
  Logical Operator : Logic  Operator=OR  AllPortsSameDT=off  OutDataTypeStr=boolean
  Logical Operator1 : Logic  AllPortsSameDT=off  OutDataTypeStr=boolean
  Switch : Switch  Criteria=u2 > Threshold
  Unit Delay : UnitDelay  SampleTime=-1  HasFrameUpgradeWarning=on
  Out1 : Outport
  wires:
  Data Type Conversion2/1 -> Logical Operator1/2
  Compare To Constant/1 -> Logical Operator1/1
  Logical Operator/1 -> Out1/1
  Constant1/1 -> Data Type Conversion1/1
  Unit Delay/1 -> Add/1
  Detect Increase/1 -> Logical Operator/2
  Logical Operator1/1 -> Logical Operator/1
  VINP_HMIZRSetTMCmd_flg/1 -> Detect Increase/1, Switch/2
  Data Type Conversion1/1 -> Add/2
  Bitwise AND/1 -> Data Type Conversion2/1
  Switch/1 -> Compare To Constant/1, Bitwise AND/1, Unit Delay/1
  Add/1 -> Switch/1
  Data Type Conversion/1 -> Switch/3
  Constant/1 -> Data Type Conversion/1

== system thc/THC/ThermalControl/AC/HMISwitchReceive4 ==
  In1 : Inport
  Add : Sum
  Bitwise AND : simulink/Logic and Bit Operations/Bitwise Operator  logicop=AND  UseBitMask=on  BitMask=bin2dec('1')  BitMaskRealWorld=Stored Integer
  Compare To Constant : simulink/Logic and Bit Operations/Compare To Constant  relop=>  const=11  OutDataTypeStr=boolean
  Constant : Constant  Value=0
  Constant1 : Constant
  Data Type Conversion : DataTypeConversion  OutDataTypeStr=uint8
  Data Type Conversion1 : DataTypeConversion  OutDataTypeStr=uint8
  Data Type Conversion2 : DataTypeConversion  OutDataTypeStr=boolean
  Detect Increase : simulink/Logic and Bit Operations/Detect Increase  vinit=0.0  OutDataTypeStr=boolean
  Logical Operator : Logic  Operator=OR  AllPortsSameDT=off  OutDataTypeStr=boolean
  Logical Operator1 : Logic  AllPortsSameDT=off  OutDataTypeStr=boolean
  Switch : Switch  Criteria=u2 > Threshold
  Unit Delay : UnitDelay  SampleTime=-1  HasFrameUpgradeWarning=on
  Out1 : Outport
  wires:
  Constant/1 -> Data Type Conversion/1
  Data Type Conversion/1 -> Switch/3
  Add/1 -> Switch/1
  Switch/1 -> Unit Delay/1, Bitwise AND/1, Compare To Constant/1
  Bitwise AND/1 -> Data Type Conversion2/1
  Data Type Conversion1/1 -> Add/2
  In1/1 -> Switch/2, Detect Increase/1
  Logical Operator1/1 -> Logical Operator/1
  Detect Increase/1 -> Logical Operator/2
  Unit Delay/1 -> Add/1
  Constant1/1 -> Data Type Conversion1/1
  Logical Operator/1 -> Out1/1
  Compare To Constant/1 -> Logical Operator1/1
  Data Type Conversion2/1 -> Logical Operator1/2

== system thc/THC/ThermalControl/AC/HMISwitchReceive5 ==
  In1 : Inport
  Add : Sum
  Bitwise AND : simulink/Logic and Bit Operations/Bitwise Operator  logicop=AND  UseBitMask=on  BitMask=bin2dec('1')  BitMaskRealWorld=Stored Integer
  Compare To Constant : simulink/Logic and Bit Operations/Compare To Constant  relop=>  const=11  OutDataTypeStr=boolean
  Constant : Constant  Value=0
  Constant1 : Constant
  Data Type Conversion : DataTypeConversion  OutDataTypeStr=uint8
  Data Type Conversion1 : DataTypeConversion  OutDataTypeStr=uint8
  Data Type Conversion2 : DataTypeConversion  OutDataTypeStr=boolean
  Detect Increase : simulink/Logic and Bit Operations/Detect Increase  vinit=0.0  OutDataTypeStr=boolean
  Logical Operator : Logic  Operator=OR  AllPortsSameDT=off  OutDataTypeStr=boolean
  Logical Operator1 : Logic  AllPortsSameDT=off  OutDataTypeStr=boolean
  Switch : Switch  Criteria=u2 > Threshold
  Unit Delay : UnitDelay  SampleTime=-1  HasFrameUpgradeWarning=on
  Out1 : Outport
  wires:
  Data Type Conversion2/1 -> Logical Operator1/2
  Compare To Constant/1 -> Logical Operator1/1
  Logical Operator/1 -> Out1/1
  Constant1/1 -> Data Type Conversion1/1
  Unit Delay/1 -> Add/1
  Detect Increase/1 -> Logical Operator/2
  Logical Operator1/1 -> Logical Operator/1
  In1/1 -> Detect Increase/1, Switch/2
  Data Type Conversion1/1 -> Add/2
  Bitwise AND/1 -> Data Type Conversion2/1
  Switch/1 -> Compare To Constant/1, Bitwise AND/1, Unit Delay/1
  Add/1 -> Switch/1
  Data Type Conversion/1 -> Switch/3
  Constant/1 -> Data Type Conversion/1

== system thc/THC/ThermalControl/AC/ModMath2 ==
  Dividend : Inport
  Divisor : Inport  Port=2
  Abs : Abs
  Constant : Constant  Value=eps
  Data Type Conversion : DataTypeConversion
  Data Type Conversion1 : DataTypeConversion
  Data Type Conversion2 : DataTypeConversion  OutDataTypeStr=single
  Divide : Product  Inputs=*/
  Equal : RelationalOperator  Operator=<=  OutDataTypeStr=boolean  RndMeth=Simplest
  Floor : Rounding
  Minus : Sum  Inputs=+-
  Product : Product
  Switch : Switch  Criteria=u2 > Threshold
  Remainder : Outport
  wires:
  Divisor/1 -> [Divisor]
  Equal/1 -> Switch/2
  Constant/1 -> Equal/2
  [Dividend] -> Divide/1
  Switch/1 -> Remainder/1
  [Dividend] -> Switch/1
  Minus/1 -> Switch/3
  Data Type Conversion2/1 -> Floor/1
  Data Type Conversion/1 -> Minus/2
  [Dividend] -> Minus/1
  Dividend/1 -> [Dividend]
  Floor/1 -> Data Type Conversion1/1
  Data Type Conversion1/1 -> Product/1
  [Divisor] -> Divide/2
  Abs/1 -> Equal/1
  [Divisor] -> Product/2
  Divide/1 -> Data Type Conversion2/1
  Product/1 -> Data Type Conversion/1
  [Divisor] -> Abs/1

== system thc/THC/ThermalControl/AC/RawdataToSettemp ==
  RawIN : Inport
  Add1 : Sum
  Constant3 : Constant  Value=0.5
  Constant4 : Constant  Value=17
  Data Type Conversion4 : DataTypeConversion  OutDataTypeStr=single
  Data Type Conversion5 : DataTypeConversion  OutDataTypeStr=single
  Data Type Conversion6 : DataTypeConversion  OutDataTypeStr=single
  Product1 : Product
  TempOut : Outport
  wires:
  RawIN/1 -> Data Type Conversion4/1
  Constant4/1 -> Data Type Conversion6/1
  Data Type Conversion6/1 -> Add1/2
  Constant3/1 -> Data Type Conversion5/1
  Data Type Conversion5/1 -> Product1/2
  Product1/1 -> Add1/1
  Add1/1 -> TempOut/1
  Data Type Conversion4/1 -> Product1/1

== system thc/THC/ThermalControl/AC/SettempToRawData ==
  TempIN : Inport
  Add : Sum  Inputs=+-
  Constant1 : Constant  Value=17
  Constant2 : Constant  Value=2
  Data Type Conversion : DataTypeConversion  OutDataTypeStr=single
  Data Type Conversion1 : DataTypeConversion  OutDataTypeStr=single
  Data Type Conversion2 : DataTypeConversion  OutDataTypeStr=single
  Data Type Conversion3 : DataTypeConversion  OutDataTypeStr=uint8
  Product : Product
  RawOut : Outport
  wires:
  Constant1/1 -> Data Type Conversion1/1
  Data Type Conversion2/1 -> Product/2
  Data Type Conversion3/1 -> RawOut/1
  Product/1 -> Data Type Conversion3/1
  Data Type Conversion1/1 -> Add/2
  TempIN/1 -> Data Type Conversion/1
  Add/1 -> Product/1
  Data Type Conversion/1 -> Add/1
  Constant2/1 -> Data Type Conversion2/1

== system thc/THC/ThermalControl/AC/Subsystem ==
  EEP_FDCFGSAirIntSta : Inport
  EEP_FDCFGSChSta : Inport  Port=2
  PwrSta : Inport  Port=3
  EEP_IONSWSta : Inport  Port=4
  FGS_AirInt_Sta : Inport  Port=5
  Compare To Constant : simulink/Logic and Bit Operations/Compare To Constant  relop===  const=0  OutDataTypeStr=boolean
  Constant1 : Constant  Value=2
  Constant10 : Constant  Value=3
  Constant{6..8,11} (4 alike) : Constant  Value=0
  Constant2 : Constant
  Constant9 : Constant
  Data Type Conversion : DataTypeConversion  OutDataTypeStr=uint8
  Data Type Conversion1 : DataTypeConversion  OutDataTypeStr=boolean
  Data Type Conversion2 : DataTypeConversion  OutDataTypeStr=boolean
  Data Type Conversion3 : DataTypeConversion  OutDataTypeStr=uint8
  Detect Change : simulink/Logic and Bit Operations/Detect Change  vinit=0  OutDataTypeStr=boolean
  Logical Operator1 : Logic  AllPortsSameDT=off  OutDataTypeStr=boolean
  Logical Operator3 : Logic  AllPortsSameDT=off  OutDataTypeStr=boolean
  Relational Operator3 : RelationalOperator  Operator=>  OutDataTypeStr=boolean  RndMeth=Simplest
  Relational Operator4 : RelationalOperator  Operator=>  OutDataTypeStr=boolean  RndMeth=Simplest
  Switch{,5..8} (5 alike) : Switch  Criteria=u2 > Threshold
  Unit Delay4 : UnitDelay  SampleTime=-1  HasFrameUpgradeWarning=on
  FGSAirIntSta : Outport
  FGSChSta : Outport  Port=2
  FGSAirIntCmd : Outport  Port=3
  FGSFuncSta : Outport  Port=4
  FGSChCmd : Outport  Port=5
  FDC_FGS_IONSW_Sta : Outport  Port=6
  FDC_FGS_ION_Cmd : Outport  Port=7
  wires:
  Constant2/1 -> Data Type Conversion3/1
  Data Type Conversion3/1 -> Switch/3
  Constant1/1 -> Data Type Conversion/1
  Data Type Conversion/1 -> Switch/1
  Logical Operator3/1 -> [PwrON]
  [FGSEnable] -> Logical Operator3/2
  Switch7/1 -> Unit Delay4/1, [FGSEnable]
  Unit Delay4/1 -> Switch8/3
  EEP_FDCFGSChSta/1 -> FGSChSta/1, Switch6/1, Detect Change/1
  Detect Change/1 -> Switch8/2
  Constant11/1 -> Data Type Conversion2/1
  Data Type Conversion2/1 -> Switch8/1
  Switch8/1 -> Switch7/3
  Data Type Conversion1/1 -> Switch7/1
  Constant9/1 -> Data Type Conversion1/1
  Compare To Constant/1 -> Switch7/2
  Logical Operator1/1 -> FDC_FGS_ION_Cmd/1
  Relational Operator4/1 -> Logical Operator1/2, Logical Operator3/1
  EEP_IONSWSta/1 -> FDC_FGS_IONSW_Sta/1, Logical Operator1/1
  Switch/1 -> FGSFuncSta/1
  Constant6/1 -> Switch5/3
  [PwrON] -> Switch6/2
  Switch5/1 -> FGSAirIntCmd/1, Relational Operator3/1
  Switch6/1 -> FGSChCmd/1
  Constant10/1 -> Relational Operator4/2
  [PwrON] -> Switch5/2
  Relational Operator3/1 -> Switch/2
  FGS_AirInt_Sta/1 -> Compare To Constant/1
  PwrSta/1 -> Relational Operator4/1
  Constant7/1 -> Relational Operator3/2
  EEP_FDCFGSAirIntSta/1 -> FGSAirIntSta/1, Switch5/1
  Constant8/1 -> Switch6/3

== system thc/THC/ThermalControl/AC/Subsystem1 ==
  Load : Inport
  DataIn : Inport  Port=2
  Switch34 : Switch  Criteria=u2 > Threshold
  Unit Delay14 : UnitDelay  SampleTime=-1  HasFrameUpgradeWarning=on
  DataOut : Outport
  wires:
  DataIn/1 -> Switch34/3
  Unit Delay14/1 -> Switch34/1
  Load/1 -> Switch34/2
  Switch34/1 -> DataOut/1, Unit Delay14/1

== system thc/THC/ThermalControl/AC/Subsystem10 ==
  Load : Inport
  DataIn : Inport  Port=2
  Switch34 : Switch  Criteria=u2 > Threshold
  Unit Delay14 : UnitDelay  SampleTime=-1  HasFrameUpgradeWarning=on
  DataOut : Outport
  wires:
  Switch34/1 -> Unit Delay14/1, DataOut/1
  Load/1 -> Switch34/2
  Unit Delay14/1 -> Switch34/1
  DataIn/1 -> Switch34/3

== system thc/THC/ThermalControl/AC/Subsystem11 ==
  Load : Inport
  DataIn : Inport  Port=2
  Switch34 : Switch  Criteria=u2 > Threshold
  Unit Delay14 : UnitDelay  SampleTime=-1  HasFrameUpgradeWarning=on
  DataOut : Outport
  wires:
  DataIn/1 -> Switch34/3
  Unit Delay14/1 -> Switch34/1
  Load/1 -> Switch34/2
  Switch34/1 -> DataOut/1, Unit Delay14/1

== system thc/THC/ThermalControl/AC/Subsystem12 ==
  Load : Inport
  DataIn : Inport  Port=2
  Switch34 : Switch  Criteria=u2 > Threshold
  Unit Delay14 : UnitDelay  SampleTime=-1  HasFrameUpgradeWarning=on
  DataOut : Outport
  wires:
  Switch34/1 -> Unit Delay14/1, DataOut/1
  Load/1 -> Switch34/2
  Unit Delay14/1 -> Switch34/1
  DataIn/1 -> Switch34/3

== system thc/THC/ThermalControl/AC/Subsystem13 ==
  Load : Inport
  DataIn : Inport  Port=2
  Switch34 : Switch  Criteria=u2 > Threshold
  Unit Delay14 : UnitDelay  SampleTime=-1  HasFrameUpgradeWarning=on
  DataOut : Outport
  wires:
  DataIn/1 -> Switch34/3
  Unit Delay14/1 -> Switch34/1
  Load/1 -> Switch34/2
  Switch34/1 -> DataOut/1, Unit Delay14/1

== system thc/THC/ThermalControl/AC/Subsystem14 ==
  Load : Inport
  DataIn : Inport  Port=2
  Switch34 : Switch  Criteria=u2 > Threshold
  Unit Delay14 : UnitDelay  SampleTime=-1  HasFrameUpgradeWarning=on
  DataOut : Outport
  wires:
  Switch34/1 -> Unit Delay14/1, DataOut/1
  Load/1 -> Switch34/2
  Unit Delay14/1 -> Switch34/1
  DataIn/1 -> Switch34/3

== system thc/THC/ThermalControl/AC/Subsystem15 ==
  Load : Inport
  DataIn : Inport  Port=2
  Switch34 : Switch  Criteria=u2 > Threshold
  Unit Delay14 : UnitDelay  SampleTime=-1  HasFrameUpgradeWarning=on
  DataOut : Outport
  wires:
  DataIn/1 -> Switch34/3
  Unit Delay14/1 -> Switch34/1
  Load/1 -> Switch34/2
  Switch34/1 -> DataOut/1, Unit Delay14/1

== system thc/THC/ThermalControl/AC/Subsystem16 ==
  Load : Inport
  DataIn : Inport  Port=2
  Switch34 : Switch  Criteria=u2 > Threshold
  Unit Delay14 : UnitDelay  SampleTime=-1  HasFrameUpgradeWarning=on
  DataOut : Outport
  wires:
  Switch34/1 -> Unit Delay14/1, DataOut/1
  Load/1 -> Switch34/2
  Unit Delay14/1 -> Switch34/1
  DataIn/1 -> Switch34/3

== system thc/THC/ThermalControl/AC/Subsystem17 ==
  Load : Inport
  DataIn : Inport  Port=2
  Switch34 : Switch  Criteria=u2 > Threshold
  Unit Delay14 : UnitDelay  SampleTime=-1  HasFrameUpgradeWarning=on
  DataOut : Outport
  wires:
  DataIn/1 -> Switch34/3
  Unit Delay14/1 -> Switch34/1
  Load/1 -> Switch34/2
  Switch34/1 -> DataOut/1, Unit Delay14/1

== system thc/THC/ThermalControl/AC/Subsystem18 ==
  Load : Inport
  DataIn : Inport  Port=2
  Switch34 : Switch  Criteria=u2 > Threshold
  Unit Delay14 : UnitDelay  SampleTime=-1  HasFrameUpgradeWarning=on
  DataOut : Outport
  wires:
  Switch34/1 -> Unit Delay14/1, DataOut/1
  Load/1 -> Switch34/2
  Unit Delay14/1 -> Switch34/1
  DataIn/1 -> Switch34/3

== system thc/THC/ThermalControl/AC/Subsystem19 ==
  Load : Inport
  DataIn : Inport  Port=2
  Switch34 : Switch  Criteria=u2 > Threshold
  Unit Delay14 : UnitDelay  SampleTime=-1  HasFrameUpgradeWarning=on
  DataOut : Outport
  wires:
  Switch34/1 -> Unit Delay14/1, DataOut/1
  Load/1 -> Switch34/2
  Unit Delay14/1 -> Switch34/1
  DataIn/1 -> Switch34/3

== system thc/THC/ThermalControl/AC/Subsystem2 ==
  Load : Inport
  DataIn : Inport  Port=2
  Switch34 : Switch  Criteria=u2 > Threshold
  Unit Delay14 : UnitDelay  SampleTime=-1  HasFrameUpgradeWarning=on
  DataOut : Outport
  wires:
  Switch34/1 -> Unit Delay14/1, DataOut/1
  Load/1 -> Switch34/2
  Unit Delay14/1 -> Switch34/1
  DataIn/1 -> Switch34/3

== system thc/THC/ThermalControl/AC/Subsystem20 ==
  Load : Inport
  DataIn : Inport  Port=2
  Switch34 : Switch  Criteria=u2 > Threshold
  Unit Delay14 : UnitDelay  SampleTime=-1  HasFrameUpgradeWarning=on
  DataOut : Outport
  wires:
  DataIn/1 -> Switch34/3
  Unit Delay14/1 -> Switch34/1
  Load/1 -> Switch34/2
  Switch34/1 -> DataOut/1, Unit Delay14/1

== system thc/THC/ThermalControl/AC/Subsystem21 ==
  Load : Inport
  DataIn : Inport  Port=2
  Switch34 : Switch  Criteria=u2 > Threshold
  Unit Delay14 : UnitDelay  SampleTime=-1  HasFrameUpgradeWarning=on
  DataOut : Outport
  wires:
  Switch34/1 -> Unit Delay14/1, DataOut/1
  Load/1 -> Switch34/2
  Unit Delay14/1 -> Switch34/1
  DataIn/1 -> Switch34/3

== system thc/THC/ThermalControl/AC/Subsystem22 ==
  Load : Inport
  DataIn : Inport  Port=2
  Switch34 : Switch  Criteria=u2 > Threshold
  Unit Delay14 : UnitDelay  SampleTime=-1  HasFrameUpgradeWarning=on
  DataOut : Outport
  wires:
  DataIn/1 -> Switch34/3
  Unit Delay14/1 -> Switch34/1
  Load/1 -> Switch34/2
  Switch34/1 -> DataOut/1, Unit Delay14/1

== system thc/THC/ThermalControl/AC/Subsystem23 ==
  Load : Inport
  DataIn : Inport  Port=2
  Switch34 : Switch  Criteria=u2 > Threshold
  Unit Delay14 : UnitDelay  SampleTime=-1  HasFrameUpgradeWarning=on
  DataOut : Outport
  wires:
  Switch34/1 -> Unit Delay14/1, DataOut/1
  Load/1 -> Switch34/2
  Unit Delay14/1 -> Switch34/1
  DataIn/1 -> Switch34/3

== system thc/THC/ThermalControl/AC/Subsystem24 ==
  Load : Inport
  DataIn : Inport  Port=2
  Switch34 : Switch  Criteria=u2 > Threshold
  Unit Delay14 : UnitDelay  SampleTime=-1  HasFrameUpgradeWarning=on
  DataOut : Outport
  wires:
  DataIn/1 -> Switch34/3
  Unit Delay14/1 -> Switch34/1
  Load/1 -> Switch34/2
  Switch34/1 -> DataOut/1, Unit Delay14/1

== system thc/THC/ThermalControl/AC/Subsystem25 ==
  Load : Inport
  DataIn : Inport  Port=2
  Switch34 : Switch  Criteria=u2 > Threshold
  Unit Delay14 : UnitDelay  SampleTime=-1  HasFrameUpgradeWarning=on
  DataOut : Outport
  wires:
  Switch34/1 -> Unit Delay14/1, DataOut/1
  Load/1 -> Switch34/2
  Unit Delay14/1 -> Switch34/1
  DataIn/1 -> Switch34/3

== system thc/THC/ThermalControl/AC/Subsystem26 ==
  Load : Inport
  DataIn : Inport  Port=2
  Switch34 : Switch  Criteria=u2 > Threshold
  Unit Delay14 : UnitDelay  SampleTime=-1  HasFrameUpgradeWarning=on
  DataOut : Outport
  wires:
  DataIn/1 -> Switch34/3
  Unit Delay14/1 -> Switch34/1
  Load/1 -> Switch34/2
  Switch34/1 -> DataOut/1, Unit Delay14/1
